simulink library "s2ss"  (R2015a)
settings: Solver=ode45  StartTime=0.0  StopTime=10.0  RelTol=1e-3
undefined symbols (not defined in the file or in its folder): AXI4, Lite
undefined symbols (not defined in the file): test
libraries: xbsIndex_r4 x92, s2ss x4
settings Model: Creator=ACS  LastModifiedBy=ACS

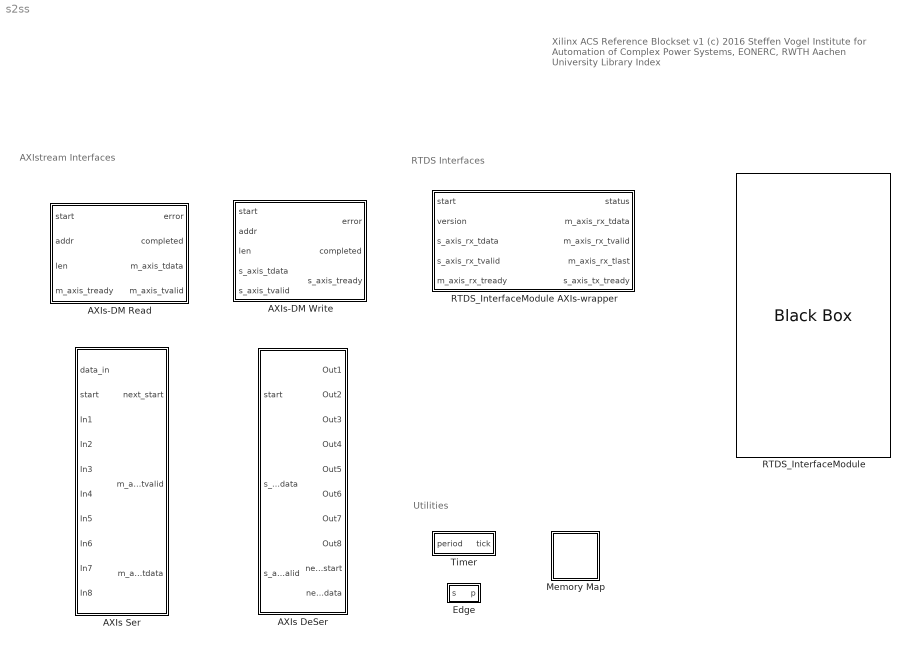
== system s2ss ==
  note: RTDS Interfaces
  note: AXIstream Interfaces
  note: Utilities
  note: Xilinx  ACS Reference Blockset v1
      | (c) 2016 Steffen Vogel
      | Institute for Automation of Complex Power Systems,
      | EONERC, RWTH Aachen University
      |
      | Library Index
  AXIs DeSer : Subsystem  mask(De-Serializing data to AXI-Steram){}
  AXIs Ser : Subsystem  mask(Serializing data to AXI-Steram){}
  AXIs-DM Read : Subsystem  mask(AXI DataMover: MM2S){}
  AXIs-DM Write : Subsystem  mask(AXI DataMover: S2MM){}
  Edge : Subsystem  mask(Rising edge detector){}
  Memory Map : Subsystem  InitFcn=|  mask(S2SS Memory Map){version=1.0, author=Steffen Vogel <stvogel@eonerc.rwth-aachen.de>, desc=System Generator Model, company_url=http://www.acs.eonerc.rwth-aachen.de, vendor=acs.eonerc.rwth-aachen.de, vendor_display_name=Institute for Automation of Complex Power Systems, EONERC, RWTH Aachen University, MaskMapDescription=test, map=[], created=[]}
      | map = xsg_memory_map();
      | %ts = floor(java.lang.System.currentTimeMillis / 1000);
      | 
      | set_param(gcb, 'map', mat2str(map));
      | %set_param(gcb, 'created', int2str(ts));
      mask prompts: desc "Description"; company_url "Company URL"; vendor_display_name "Vendor Display Name"
      mask help:
      | - This ROM contains a encoded memory map of all
      | Gateway In / Out blocks with an AXI4-Lite interface implementation.
      |
      | - The memory map is encoded in the function xsg_memory_map().
      |
      | - The CPU has to read the memory map word by word by using control
      |   registers 'map_addr' and 'map_data':
      |      1. Write address to 0x0 (map_addr)
      |      2. Read word from 0x4 (map_data)
      |      3. Increment address by 1 and start from 1
      |      4. Stop if word == 0xDEADBABE
      mask init:
      | set_param(gcb, 'MaskMapDescription', 'test');
      mask DialogControl DescTextMapVar Prompt: %<MaskMapDescription>
      mask Display:
      | color = [ hex2dec('FF') hex2dec('19') hex2dec('19') ] ./ 255;
      | 
      | patch([ 0 1 1 0 ], [ 0 0 0.2 0.2 ], color);
      | patch([ 0 1 1 0 ], [ 0.4 0.4 0.6 0.6 ], color);
      | patch([ 0 1 1 0 ], [ 0.8 0.8 1 1 ], color);
  RTDS_InterfaceModule : xbsIndex_r4/Black Box  init_code=RTDS_InterfaceModule_config  sim_method=ISE Simulator  verbose=off  block_type=blackbox2
  RTDS_InterfaceModule AXIs-wrapper : Subsystem  mask(AXI-Stream wrapper for RTDS_InterfaceModule blackbox){}
      mask Display: image(imread('logos/rtds.png'), [ 0.3 0.5 0.4 0.4 ])
  Timer : Subsystem  mask(Generate ticks every period cycles){}

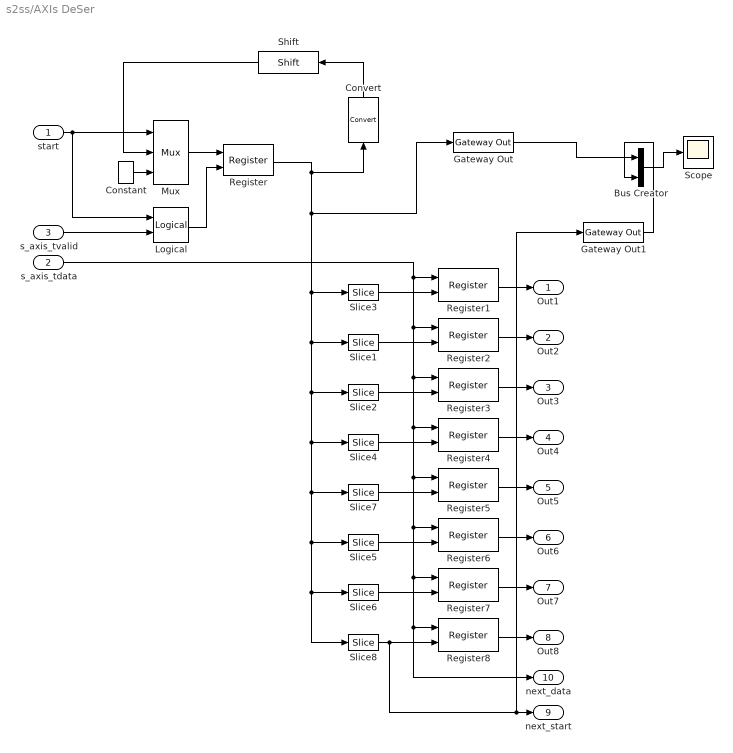
== system s2ss/AXIs DeSer ==
  start : Inport
  s_axis_tdata : Inport  Port=2
  s_axis_tvalid : Inport  Port=3
  Bus Creator : BusCreator  Inputs=2
  Constant : xbsIndex_r4/Constant  const=1  gui_display_data_type=Fixed-point  arith_type=Unsigned  n_bits=8  bin_pt=0  preci_type=Single  exp_width=8  frac_width=24  explicit_period=off  period=1  equ=P=C  opselect=C  inp2=PCIN>>17  opr=+  inp1=P  carry=CIN  dbl_ovrd=off  block_type=constant
  Convert : xbsIndex_r4/Convert  gui_display_data_type=Fixed-point  arith_type="Signed  (2's comp)"  n_bits=8  bin_pt=0  float_type=Single  exp_bits=8  fraction_bits=24  quantization=Truncate  overflow=Wrap  en=off  latency=0  pipeline=off  dbl_ovrd=off  block_type=convert
  Gateway Out : xbsIndex_r4/Gateway Out  inherit_from_input=off  hdl_port=on  rows=1  columns=1  UseAsDAC=off  DACChannel='1'  interface=None  automatic_assignment=on  address_offset=hex2dec('00')  intf_name=''  intf_description=''  timing_constraint=None  locs_specified=off  LOCs={}  io_standard={}  block_type=gatewayout
  Gateway Out1 : xbsIndex_r4/Gateway Out  inherit_from_input=off  hdl_port=on  rows=1  columns=1  UseAsDAC=off  DACChannel='1'  interface=None  automatic_assignment=on  address_offset=hex2dec('00')  intf_name=''  intf_description=''  timing_constraint=None  locs_specified=off  LOCs={}  io_standard={}  block_type=gatewayout
  Logical : xbsIndex_r4/Logical  logical_function=OR  inputs=2  en=off  latency=0  precision=Full  arith_type=Unsigned  n_bits=16  bin_pt=0  align_bp=on  dbl_ovrd=off  block_type=logical
  Mux : xbsIndex_r4/Mux  inputs=2  en=off  latency=0  precision=User Defined  arith_type=Unsigned  n_bits=8  bin_pt=0  quantization=Truncate  overflow=Wrap  dbl_ovrd=off  block_type=mux
  Register : xbsIndex_r4/Register  init=0  rst=off  en=on  dbl_ovrd=off  block_type=register
  Register{1..8} (8 alike) : xbsIndex_r4/Register  init=1  rst=off  en=on  dbl_ovrd=off  block_type=register
  Scope : Scope
  Shift : xbsIndex_r4/Shift  shift_dir=Left  shift_bits=1  en=off  latency=0  precision=Full  arith_type="Signed  (2's comp)"  n_bits=16  bin_pt=14  quantization=Truncate  overflow=Wrap  dbl_ovrd=off  block_type=shift
  Slice1 : xbsIndex_r4/Slice  nbits=1  boolean_output=on  mode=Lower Bit Location + Width  bit1=0  base1=MSB of Input  bit0=1  base0=LSB of Input  dbl_ovrd=off  block_type=slice
  Slice2 : xbsIndex_r4/Slice  nbits=1  boolean_output=on  mode=Lower Bit Location + Width  bit1=0  base1=MSB of Input  bit0=2  base0=LSB of Input  dbl_ovrd=off  block_type=slice
  Slice3 : xbsIndex_r4/Slice  nbits=1  boolean_output=on  mode=Lower Bit Location + Width  bit1=0  base1=MSB of Input  bit0=0  base0=LSB of Input  dbl_ovrd=off  block_type=slice
  Slice4 : xbsIndex_r4/Slice  nbits=1  boolean_output=on  mode=Lower Bit Location + Width  bit1=0  base1=MSB of Input  bit0=3  base0=LSB of Input  dbl_ovrd=off  block_type=slice
  Slice5 : xbsIndex_r4/Slice  nbits=1  boolean_output=on  mode=Lower Bit Location + Width  bit1=0  base1=MSB of Input  bit0=5  base0=LSB of Input  dbl_ovrd=off  block_type=slice
  Slice6 : xbsIndex_r4/Slice  nbits=1  boolean_output=on  mode=Lower Bit Location + Width  bit1=0  base1=MSB of Input  bit0=6  base0=LSB of Input  dbl_ovrd=off  block_type=slice
  Slice7 : xbsIndex_r4/Slice  nbits=1  boolean_output=on  mode=Lower Bit Location + Width  bit1=0  base1=MSB of Input  bit0=4  base0=LSB of Input  dbl_ovrd=off  block_type=slice
  Slice8 : xbsIndex_r4/Slice  nbits=1  boolean_output=on  mode=Lower Bit Location + Width  bit1=0  base1=MSB of Input  bit0=7  base0=LSB of Input  dbl_ovrd=off  block_type=slice
  Out1 : Outport
  Out2 : Outport  Port=2
  Out3 : Outport  Port=3
  Out4 : Outport  Port=4
  Out5 : Outport  Port=5
  Out6 : Outport  Port=6
  Out7 : Outport  Port=7
  Out8 : Outport  Port=8
  next_start : Outport  Port=9
  next_data : Outport  Port=10
  wires:
  Gateway Out1/1 -> Bus Creator/2
  Gateway Out/1 -> Bus Creator/1
  Bus Creator/1 -> Scope/1
  Shift/1 -> Mux/2
  Constant/1 -> Mux/3
  Logical/1 -> Register/2
  s_axis_tvalid/1 -> Logical/2
  Mux/1 -> Register/1
  start/1 -> Mux/1, Logical/1
  Convert/1 -> Shift/1
  Register8/1 -> Out8/1
  Slice8/1 -> next_start/1, Gateway Out1/1, Register8/2
  Register7/1 -> Out7/1
  Slice6/1 -> Register7/2
  Register6/1 -> Out6/1
  Slice5/1 -> Register6/2
  Register5/1 -> Out5/1
  Slice7/1 -> Register5/2
  Register4/1 -> Out4/1
  Slice4/1 -> Register4/2
  Register3/1 -> Out3/1
  Slice2/1 -> Register3/2
  Register2/1 -> Out2/1
  Slice1/1 -> Register2/2
  Register1/1 -> Out1/1
  s_axis_tdata/1 -> Register1/1, Register8/1, next_data/1, Register7/1, Register6/1, Register5/1, Register4/1, Register3/1, Register2/1
  Register/1 -> Convert/1, Slice3/1, Slice1/1, Slice2/1, Slice4/1, Slice7/1, Slice5/1, Slice6/1, Slice8/1, Gateway Out/1
  Slice3/1 -> Register1/2

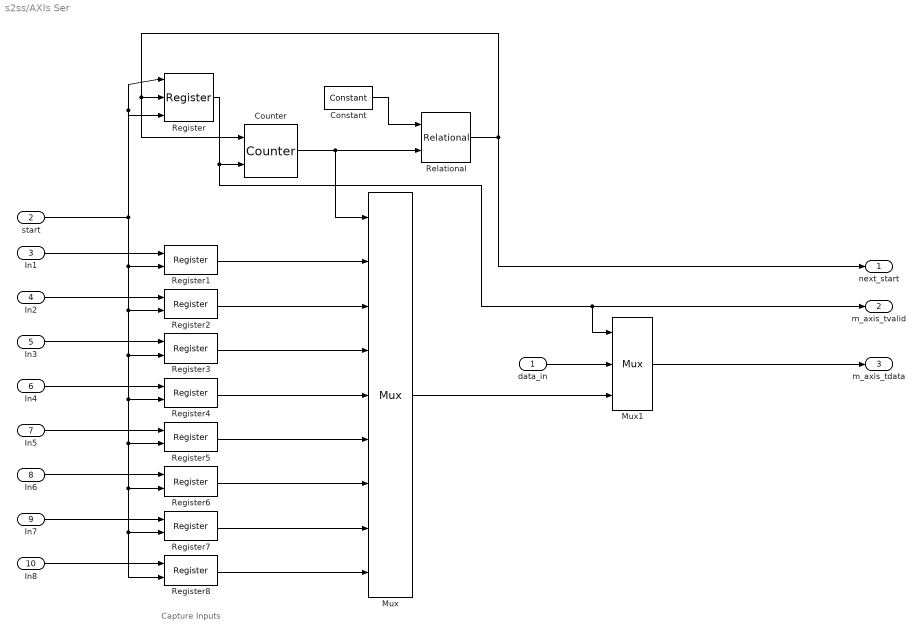
== system s2ss/AXIs Ser ==
  note: Capture Inputs
  data_in : Inport
  start : Inport  Port=2
  In1 : Inport  Port=3
  In2 : Inport  Port=4
  In3 : Inport  Port=5
  In4 : Inport  Port=6
  In5 : Inport  Port=7
  In6 : Inport  Port=8
  In7 : Inport  Port=9
  In8 : Inport  Port=10
  Constant : xbsIndex_r4/Constant  const=7  gui_display_data_type=Fixed-point  arith_type=Unsigned  n_bits=3  bin_pt=0  preci_type=Single  exp_width=8  frac_width=24  explicit_period=off  period=1  equ=P=C  opselect=C  inp2=PCIN>>17  opr=+  inp1=P  carry=CIN  dbl_ovrd=off  block_type=constant
  Counter : xbsIndex_r4/Counter  cnt_type=Free Running  cnt_to=Inf  operation=Up  start_count=0  cnt_by_val=1  arith_type=Unsigned  n_bits=3  bin_pt=0  load_pin=off  rst=on  en=on  explicit_period=on  period=1  use_behavioral_HDL=off  implementation=Fabric  dbl_ovrd=off  block_type=counter
  Mux : xbsIndex_r4/Mux  inputs=8  en=off  latency=0  precision=Full  arith_type=Unsigned  n_bits=16  bin_pt=14  quantization=Truncate  overflow=Wrap  dbl_ovrd=off  block_type=mux
  Mux1 : xbsIndex_r4/Mux  inputs=2  en=off  latency=1  precision=Full  arith_type=Unsigned  n_bits=16  bin_pt=14  quantization=Truncate  overflow=Wrap  dbl_ovrd=off  block_type=mux
  Register : xbsIndex_r4/Register  init=0  rst=on  en=on  dbl_ovrd=off  block_type=register
  Register{1..8} (8 alike) : xbsIndex_r4/Register  init=1  rst=off  en=on  dbl_ovrd=off  block_type=register
  Relational : xbsIndex_r4/Relational  mode=a=b  op_type=Bool  en=off  latency=0  dbl_ovrd=off  block_type=relational
  next_start : Outport
  "m_axis_tvalid " : Outport  Port=2
  m_axis_tdata : Outport  Port=3
  wires:
  data_in/1 -> Mux1/2
  Mux1/1 -> m_axis_tdata/1
  Register/1 -> "m_axis_tvalid "/1, Mux1/1, Counter/2
  Relational/1 -> next_start/1, Register/2, Counter/1
  Constant/1 -> Relational/1
  Register8/1 -> Mux/9
  Register7/1 -> Mux/8
  Register6/1 -> Mux/7
  Register5/1 -> Mux/6
  Register4/1 -> Mux/5
  Register3/1 -> Mux/4
  Register2/1 -> Mux/3
  Register1/1 -> Mux/2
  Counter/1 -> Relational/2, Mux/1
  Mux/1 -> Mux1/3
  In8/1 -> Register8/1
  In7/1 -> Register7/1
  In6/1 -> Register6/1
  In5/1 -> Register5/1
  In4/1 -> Register4/1
  In1/1 -> Register1/1
  In2/1 -> Register2/1
  In3/1 -> Register3/1
  start/1 -> Register1/2, Register2/2, Register3/2, Register4/2, Register5/2, Register6/2, Register7/2, Register8/2, Register/1, Register/3

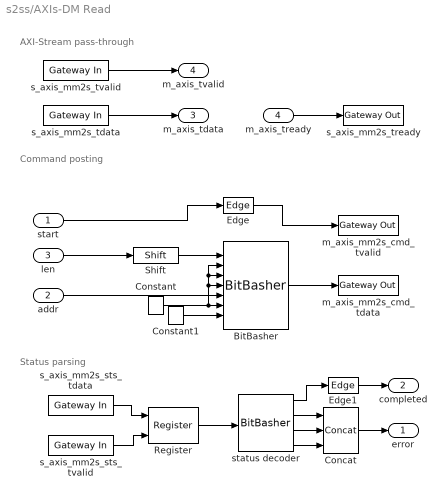
== system s2ss/AXIs-DM Read ==
  note: AXI-Stream pass-through
  note: Command posting
  note: Status parsing
  start : Inport
  addr : Inport  Port=2
  len : Inport  Port=3
  m_axis_tready : Inport  Port=4
  "BitBasher " : xbsIndex_r4/BitBasher  bitexpr=cmd={4'h0,tag[3:0],saddr[31:0],drr[0],eof[0],dsa[5:0],type[0],btt[22:0]}  display_expr=off  sr_1=cmd  arith_type1=Unsigned  bin_pt1=0  sr_2=2  arith_type2=Unsigned  bin_pt2=0  sr_3=3  arith_type3=Unsigned  bin_pt3=0  sr_4=4  arith_type4=Unsigned  bin_pt4=0  dbl_ovrd=off  block_type=bitbasher
  Concat : xbsIndex_r4/Concat  num_inputs=3  dbl_ovrd=off  block_type=concat
  Constant : xbsIndex_r4/Constant  const=0  gui_display_data_type=Fixed-point  arith_type=Unsigned  n_bits=16  bin_pt=0  preci_type=Single  exp_width=8  frac_width=24  explicit_period=off  period=1  equ=P=C  opselect=C  inp2=PCIN>>17  opr=+  inp1=P  carry=CIN  dbl_ovrd=off  block_type=constant
  Constant1 : xbsIndex_r4/Constant  const=1  gui_display_data_type=Fixed-point  arith_type=Unsigned  n_bits=16  bin_pt=0  preci_type=Single  exp_width=8  frac_width=24  explicit_period=off  period=1  equ=P=C  opselect=C  inp2=PCIN>>17  opr=+  inp1=P  carry=CIN  dbl_ovrd=off  block_type=constant
  Edge : s2ss/Edge  SystemSampleTime=-1
  Edge1 : s2ss/Edge  SystemSampleTime=-1
  Register : xbsIndex_r4/Register  init=0  rst=off  en=on  dbl_ovrd=off  block_type=register
  Shift : xbsIndex_r4/Shift  shift_dir=Left  shift_bits=2  en=off  latency=0  precision=User Defined  arith_type=Unsigned  n_bits=23  bin_pt=0  quantization=Truncate  overflow=Wrap  dbl_ovrd=off  block_type=shift
  m_axis_mm2s_cmd_tdata : xbsIndex_r4/Gateway Out  inherit_from_input=off  hdl_port=on  rows=1  columns=1  UseAsDAC=off  DACChannel='1'  interface=None  automatic_assignment=on  address_offset=hex2dec('00')  intf_name=''  intf_description=''  timing_constraint=None  locs_specified=off  LOCs={}  io_standard={}  block_type=gatewayout
  m_axis_mm2s_cmd_tvalid : xbsIndex_r4/Gateway Out  inherit_from_input=off  hdl_port=on  rows=1  columns=1  UseAsDAC=off  DACChannel='1'  interface=None  automatic_assignment=on  address_offset=hex2dec('00')  intf_name=''  intf_description=''  timing_constraint=None  locs_specified=off  LOCs={}  io_standard={}  block_type=gatewayout
  s_axis_mm2s_sts_tdata : xbsIndex_r4/Gateway In  gui_display_data_type=Fixed-point  arith_type=Unsigned  n_bits=8  bin_pt=0  preci_type=Single  exp_width=8  frac_width=24  rows=1  columns=1  quantization=Truncate  overflow=Wrap  period=1  UseAsADC=off  ADCChannel='1'  interface=None  automatic_assignment=on  address_offset=hex2dec('00')  intf_name=''  intf_description=''  timing_constraint=None  locs_specified=off  LOCs={}  io_standard={}  inherit_from_input=off  hdl_port=on  dbl_ovrd=off  block_type=gatewayin
  s_axis_mm2s_sts_tvalid : xbsIndex_r4/Gateway In  gui_display_data_type=Boolean  arith_type=Boolean  n_bits=1  bin_pt=0  preci_type=Single  exp_width=8  frac_width=24  rows=1  columns=1  quantization="Round  (unbiased: +/- Inf)"  overflow=Saturate  period=1  UseAsADC=off  ADCChannel='1'  interface=None  automatic_assignment=on  address_offset=hex2dec('00')  intf_name=''  intf_description=''  timing_constraint=None  locs_specified=off  LOCs={}  io_standard={}  inherit_from_input=off  hdl_port=on  dbl_ovrd=off  block_type=gatewayin
  s_axis_mm2s_tdata : xbsIndex_r4/Gateway In  gui_display_data_type=Fixed-point  arith_type=Unsigned  n_bits=32  bin_pt=0  preci_type=Single  exp_width=8  frac_width=24  rows=1  columns=1  quantization=Truncate  overflow=Wrap  period=1  UseAsADC=off  ADCChannel='1'  interface=None  automatic_assignment=on  address_offset=hex2dec('00')  intf_name=''  intf_description=''  timing_constraint=None  locs_specified=off  LOCs={}  io_standard={}  inherit_from_input=off  hdl_port=on  dbl_ovrd=off  block_type=gatewayin
  s_axis_mm2s_tready : xbsIndex_r4/Gateway Out  inherit_from_input=off  hdl_port=on  rows=1  columns=1  UseAsDAC=off  DACChannel='1'  interface=None  automatic_assignment=on  address_offset=hex2dec('00')  intf_name=''  intf_description=''  timing_constraint=None  locs_specified=off  LOCs={}  io_standard={}  block_type=gatewayout
  s_axis_mm2s_tvalid : xbsIndex_r4/Gateway In  gui_display_data_type=Boolean  arith_type=Boolean  n_bits=16  bin_pt=14  preci_type=Single  exp_width=8  frac_width=24  rows=1  columns=1  quantization="Round  (unbiased: +/- Inf)"  overflow=Saturate  period=1  UseAsADC=off  ADCChannel='1'  interface=None  automatic_assignment=on  address_offset=hex2dec('00')  intf_name=''  intf_description=''  timing_constraint=None  locs_specified=off  LOCs={}  io_standard={}  inherit_from_input=off  hdl_port=on  dbl_ovrd=off  block_type=gatewayin
  status decoder : xbsIndex_r4/BitBasher  bitexpr=|  display_expr=off  sr_1=okay  arith_type1=Unsigned  bin_pt1=0  sr_2=slverr  arith_type2=Unsigned  bin_pt2=0  sr_3=decerr  arith_type3=Unsigned  bin_pt3=0  sr_4=interr  arith_type4=Unsigned  bin_pt4=0  dbl_ovrd=off  block_type=bitbasher
      | okay={sts[7]}
      | slverr={sts[6]}
      | decerr={sts[5]}
      | interr={sts[4]}
  error : Outport
  completed : Outport  Port=2
  m_axis_tdata : Outport  Port=3
  m_axis_tvalid : Outport  Port=4
  wires:
  Shift/1 -> "BitBasher "/1
  "BitBasher "/1 -> m_axis_mm2s_cmd_tdata/1
  s_axis_mm2s_sts_tdata/1 -> Register/1
  s_axis_mm2s_sts_tvalid/1 -> Register/2
  Register/1 -> status decoder/1
  status decoder/4 -> Concat/3
  Concat/1 -> error/1
  Edge/1 -> m_axis_mm2s_cmd_tvalid/1
  len/1 -> Shift/1
  start/1 -> Edge/1
  status decoder/3 -> Concat/2
  status decoder/2 -> Concat/1
  s_axis_mm2s_tvalid/1 -> m_axis_tvalid/1
  s_axis_mm2s_tdata/1 -> m_axis_tdata/1
  m_axis_tready/1 -> s_axis_mm2s_tready/1
  addr/1 -> "BitBasher "/5
  Constant/1 -> "BitBasher "/2, "BitBasher "/3, "BitBasher "/4, "BitBasher "/6
  status decoder/1 -> Edge1/1
  Edge1/1 -> completed/1
  Constant1/1 -> "BitBasher "/7

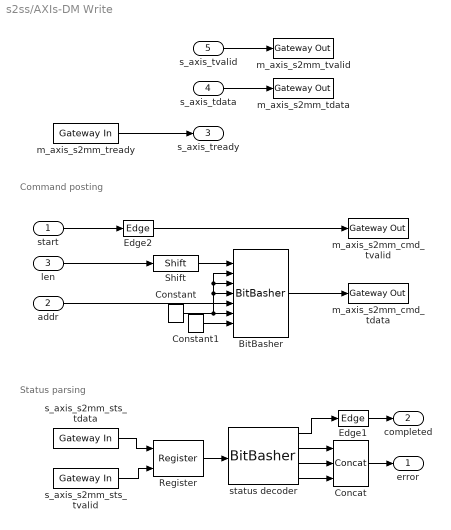
== system s2ss/AXIs-DM Write ==
  note: Command posting
  note: Status parsing
  start : Inport
  addr : Inport  Port=2
  len : Inport  Port=3
  s_axis_tdata : Inport  Port=4
  s_axis_tvalid : Inport  Port=5
  "BitBasher " : xbsIndex_r4/BitBasher  bitexpr=cmd={4'h0,tag[3:0],saddr[31:0],drr[0],eof[0],dsa[5:0],type[0],btt[22:0]}  display_expr=off  sr_1=cmd  arith_type1=Unsigned  bin_pt1=0  sr_2=2  arith_type2=Unsigned  bin_pt2=0  sr_3=3  arith_type3=Unsigned  bin_pt3=0  sr_4=4  arith_type4=Unsigned  bin_pt4=0  dbl_ovrd=off  block_type=bitbasher
  Concat : xbsIndex_r4/Concat  num_inputs=3  dbl_ovrd=off  block_type=concat
  Constant : xbsIndex_r4/Constant  const=0  gui_display_data_type=Fixed-point  arith_type=Unsigned  n_bits=16  bin_pt=0  preci_type=Single  exp_width=8  frac_width=24  explicit_period=off  period=1  equ=P=C  opselect=C  inp2=PCIN>>17  opr=+  inp1=P  carry=CIN  dbl_ovrd=off  block_type=constant
  Constant1 : xbsIndex_r4/Constant  const=1  gui_display_data_type=Fixed-point  arith_type=Unsigned  n_bits=16  bin_pt=0  preci_type=Single  exp_width=8  frac_width=24  explicit_period=off  period=1  equ=P=C  opselect=C  inp2=PCIN>>17  opr=+  inp1=P  carry=CIN  dbl_ovrd=off  block_type=constant
  Edge1 : s2ss/Edge  SystemSampleTime=-1
  Edge2 : s2ss/Edge  SystemSampleTime=-1
  Register : xbsIndex_r4/Register  init=0  rst=off  en=on  dbl_ovrd=off  block_type=register
  Shift : xbsIndex_r4/Shift  shift_dir=Left  shift_bits=2  en=off  latency=0  precision=User Defined  arith_type=Unsigned  n_bits=23  bin_pt=0  quantization=Truncate  overflow=Wrap  dbl_ovrd=off  block_type=shift
  m_axis_s2mm_cmd_tdata : xbsIndex_r4/Gateway Out  inherit_from_input=off  hdl_port=on  rows=1  columns=1  UseAsDAC=off  DACChannel='1'  interface=None  automatic_assignment=on  address_offset=hex2dec('00')  intf_name=''  intf_description=''  timing_constraint=None  locs_specified=off  LOCs={}  io_standard={}  block_type=gatewayout
  m_axis_s2mm_cmd_tvalid : xbsIndex_r4/Gateway Out  inherit_from_input=off  hdl_port=on  rows=1  columns=1  UseAsDAC=off  DACChannel='1'  interface=None  automatic_assignment=on  address_offset=hex2dec('00')  intf_name=''  intf_description=''  timing_constraint=None  locs_specified=off  LOCs={}  io_standard={}  block_type=gatewayout
  m_axis_s2mm_tdata : xbsIndex_r4/Gateway Out  inherit_from_input=off  hdl_port=on  rows=1  columns=1  UseAsDAC=off  DACChannel='1'  interface=None  automatic_assignment=on  address_offset=hex2dec('00')  intf_name=''  intf_description=''  timing_constraint=None  locs_specified=off  LOCs={}  io_standard={}  block_type=gatewayout
  m_axis_s2mm_tready : xbsIndex_r4/Gateway In  gui_display_data_type=Boolean  arith_type=Boolean  n_bits=8  bin_pt=0  preci_type=Single  exp_width=8  frac_width=24  rows=1  columns=1  quantization=Truncate  overflow=Wrap  period=1  UseAsADC=off  ADCChannel='1'  interface=None  automatic_assignment=on  address_offset=hex2dec('00')  intf_name=''  intf_description=''  timing_constraint=None  locs_specified=off  LOCs={}  io_standard={}  inherit_from_input=off  hdl_port=on  dbl_ovrd=off  block_type=gatewayin
  m_axis_s2mm_tvalid : xbsIndex_r4/Gateway Out  inherit_from_input=off  hdl_port=on  rows=1  columns=1  UseAsDAC=off  DACChannel='1'  interface=None  automatic_assignment=on  address_offset=hex2dec('00')  intf_name=''  intf_description=''  timing_constraint=None  locs_specified=off  LOCs={}  io_standard={}  block_type=gatewayout
  s_axis_s2mm_sts_tdata : xbsIndex_r4/Gateway In  gui_display_data_type=Fixed-point  arith_type=Unsigned  n_bits=8  bin_pt=0  preci_type=Single  exp_width=8  frac_width=24  rows=1  columns=1  quantization=Truncate  overflow=Wrap  period=1  UseAsADC=off  ADCChannel='1'  interface=None  automatic_assignment=on  address_offset=hex2dec('00')  intf_name=''  intf_description=''  timing_constraint=None  locs_specified=off  LOCs={}  io_standard={}  inherit_from_input=off  hdl_port=on  dbl_ovrd=off  block_type=gatewayin
  s_axis_s2mm_sts_tvalid : xbsIndex_r4/Gateway In  gui_display_data_type=Boolean  arith_type=Boolean  n_bits=16  bin_pt=14  preci_type=Single  exp_width=8  frac_width=24  rows=1  columns=1  quantization="Round  (unbiased: +/- Inf)"  overflow=Saturate  period=1  UseAsADC=off  ADCChannel='1'  interface=None  automatic_assignment=on  address_offset=hex2dec('00')  intf_name=''  intf_description=''  timing_constraint=None  locs_specified=off  LOCs={}  io_standard={}  inherit_from_input=off  hdl_port=on  dbl_ovrd=off  block_type=gatewayin
  status decoder : xbsIndex_r4/BitBasher  bitexpr=|  display_expr=off  sr_1=okay  arith_type1=Unsigned  bin_pt1=0  sr_2=slverr  arith_type2=Unsigned  bin_pt2=0  sr_3=decerr  arith_type3=Unsigned  bin_pt3=0  sr_4=interr  arith_type4=Unsigned  bin_pt4=0  dbl_ovrd=off  block_type=bitbasher
      | okay={sts[7]}
      | slverr={sts[6]}
      | decerr={sts[5]}
      | interr={sts[4]}
  error : Outport
  completed : Outport  Port=2
  s_axis_tready : Outport  Port=3
  wires:
  addr/1 -> "BitBasher "/5
  Shift/1 -> "BitBasher "/1
  "BitBasher "/1 -> m_axis_s2mm_cmd_tdata/1
  s_axis_s2mm_sts_tdata/1 -> Register/1
  s_axis_s2mm_sts_tvalid/1 -> Register/2
  Register/1 -> status decoder/1
  status decoder/4 -> Concat/3
  Concat/1 -> error/1
  start/1 -> Edge2/1
  s_axis_tvalid/1 -> m_axis_s2mm_tvalid/1
  s_axis_tdata/1 -> m_axis_s2mm_tdata/1
  len/1 -> Shift/1
  Edge2/1 -> m_axis_s2mm_cmd_tvalid/1
  m_axis_s2mm_tready/1 -> s_axis_tready/1
  status decoder/3 -> Concat/2
  status decoder/2 -> Concat/1
  status decoder/1 -> Edge1/1
  Constant/1 -> "BitBasher "/6, "BitBasher "/4, "BitBasher "/3, "BitBasher "/2
  Edge1/1 -> completed/1
  Constant1/1 -> "BitBasher "/7

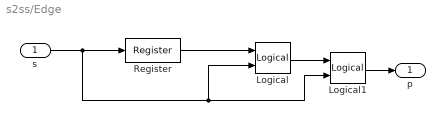
== system s2ss/Edge ==
  s : Inport
  Logical : xbsIndex_r4/Logical  logical_function=XOR  inputs=2  en=off  latency=0  precision=Full  arith_type=Unsigned  n_bits=16  bin_pt=0  align_bp=on  dbl_ovrd=off  block_type=logical
  Logical1 : xbsIndex_r4/Logical  logical_function=AND  inputs=2  en=off  latency=0  precision=Full  arith_type=Unsigned  n_bits=16  bin_pt=0  align_bp=on  dbl_ovrd=off  block_type=logical
  Register : xbsIndex_r4/Register  init=0  rst=off  en=off  dbl_ovrd=off  block_type=register
  p : Outport
  wires:
  s/1 -> Logical/2, Logical1/2, Register/1
  Register/1 -> Logical/1
  Logical1/1 -> p/1
  Logical/1 -> Logical1/1

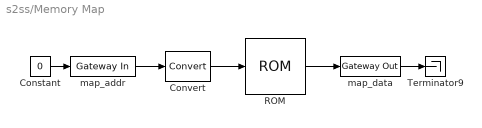
== system s2ss/Memory Map ==
  Constant : Constant  Value=0
  Convert : xbsIndex_r4/Convert  gui_display_data_type=Fixed-point  arith_type=Unsigned  n_bits=ceil(log2(length(map)))  bin_pt=0  float_type=Single  exp_bits=8  fraction_bits=24  quantization=Truncate  overflow=Wrap  en=off  latency=1  pipeline=off  dbl_ovrd=off  block_type=convert
  ROM : xbsIndex_r4/ROM  depth=length(map)  initVector=map  distributed_mem=Block RAM  rst=off  init_reg=0  en=off  latency=1  gui_display_data_type=Fixed-point  arith_type=Unsigned  n_bits=32  bin_pt=0  preci_type=Single  exp_width=8  frac_width=24  optimize=Area  use_rpm=on  dbl_ovrd=off  block_type=sprom
  Terminator9 : Terminator
  map_addr : xbsIndex_r4/Gateway In  gui_display_data_type=Fixed-point  arith_type=Unsigned  n_bits=32  bin_pt=0  preci_type=Single  exp_width=8  frac_width=24  rows=1  columns=1  quantization=Truncate  overflow=Wrap  period=1  UseAsADC=off  ADCChannel='1'  interface=AXI4-Lite  automatic_assignment=off  address_offset=hex2dec('00')  intf_name=''  intf_description=''  timing_constraint=None  locs_specified=off  LOCs={}  io_standard={}  inherit_from_input=off  hdl_port=on  dbl_ovrd=off  block_type=gatewayin
  map_data : xbsIndex_r4/Gateway Out  inherit_from_input=off  hdl_port=on  rows=1  columns=1  UseAsDAC=off  DACChannel='1'  interface=AXI4-Lite  automatic_assignment=off  address_offset=hex2dec('04')  intf_name=''  intf_description=''  timing_constraint=None  locs_specified=off  LOCs={}  io_standard={}  block_type=gatewayout
  wires:
  ROM/1 -> map_data/1
  map_addr/1 -> Convert/1
  Convert/1 -> ROM/1
  map_data/1 -> Terminator9/1
  Constant/1 -> map_addr/1

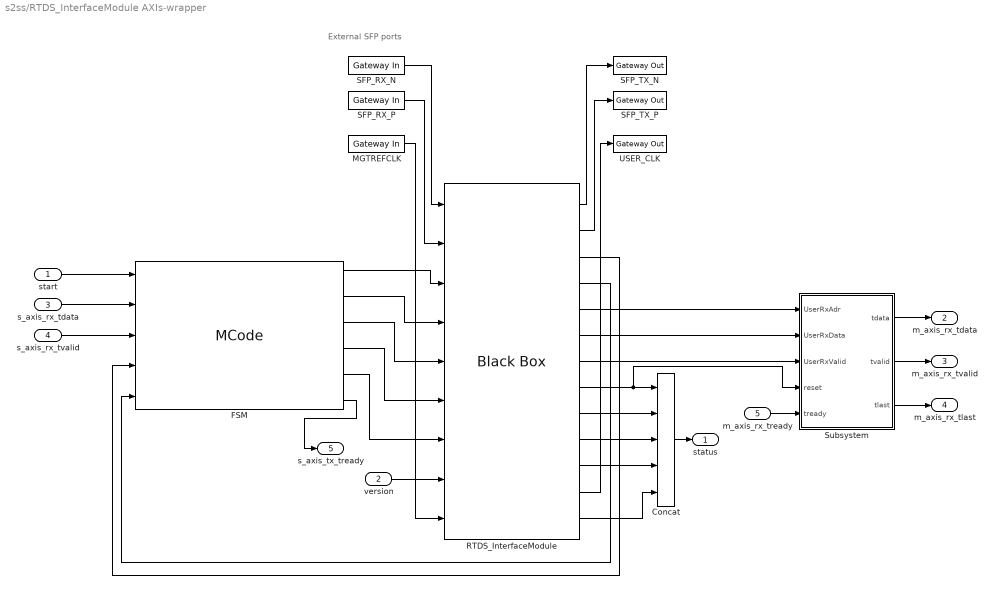
== system s2ss/RTDS_InterfaceModule AXIs-wrapper ==
  note: External SFP ports
  start : Inport
  version : Inport  Port=2
  s_axis_rx_tdata : Inport  Port=3
  s_axis_rx_tvalid : Inport  Port=4
  m_axis_rx_tready : Inport  Port=5
  Concat : xbsIndex_r4/Concat  num_inputs=5  dbl_ovrd=off  block_type=concat
  FSM : xbsIndex_r4/MCode  mfname=RTDS_InferfaceModule_fsm  explicit_period=off  period=1  inputsTable={'boundInpExpr'=>['','','',''],'inputs'=>['start','NbValues','UserTxFull','UserTxInProgress']}  outputsTable={'outputs'=>['UserTxAdr','UserTxData','UserTxWr','UserLockBank','UserFreeBank'],'suppressOut'=>['off','off','off','off','off']}  enable_stdout=off  enable_debug=off  suppress_output=on  defparams={}  hide_port_list={}  dbl_ovrd=off  block_type=mcode
  MGTREFCLK : xbsIndex_r4/Gateway In  gui_display_data_type=Boolean  arith_type=Boolean  n_bits=16  bin_pt=14  preci_type=Single  exp_width=8  frac_width=24  rows=1  columns=1  quantization="Round  (unbiased: +/- Inf)"  overflow=Saturate  period=1  UseAsADC=off  ADCChannel='1'  interface=None  automatic_assignment=on  address_offset=hex2dec('00')  intf_name=''  intf_description=''  timing_constraint=None  locs_specified=off  LOCs={}  io_standard={}  inherit_from_input=off  hdl_port=on  dbl_ovrd=off  block_type=gatewayin
  RTDS_InterfaceModule : xbsIndex_r4/Black Box  init_code=RTDS_InterfaceModule_config  sim_method=ISE Simulator  verbose=off  block_type=blackbox2
  SFP_RX_N : xbsIndex_r4/Gateway In  gui_display_data_type=Boolean  arith_type=Boolean  n_bits=1  bin_pt=0  preci_type=Single  exp_width=8  frac_width=24  rows=1  columns=1  quantization="Round  (unbiased: +/- Inf)"  overflow=Saturate  period=1  UseAsADC=off  ADCChannel='1'  interface=None  automatic_assignment=on  address_offset=hex2dec('00')  intf_name=''  intf_description=''  timing_constraint=None  locs_specified=off  LOCs={}  io_standard={}  inherit_from_input=off  hdl_port=on  dbl_ovrd=off  block_type=gatewayin
  SFP_RX_P : xbsIndex_r4/Gateway In  gui_display_data_type=Boolean  arith_type=Boolean  n_bits=16  bin_pt=14  preci_type=Single  exp_width=8  frac_width=24  rows=1  columns=1  quantization="Round  (unbiased: +/- Inf)"  overflow=Saturate  period=1  UseAsADC=off  ADCChannel='1'  interface=None  automatic_assignment=on  address_offset=hex2dec('00')  intf_name=''  intf_description=''  timing_constraint=None  locs_specified=off  LOCs={}  io_standard={}  inherit_from_input=off  hdl_port=on  dbl_ovrd=off  block_type=gatewayin
  SFP_TX_N : xbsIndex_r4/Gateway Out  inherit_from_input=off  hdl_port=on  rows=1  columns=1  UseAsDAC=off  DACChannel='1'  interface=None  automatic_assignment=on  address_offset=hex2dec('00')  intf_name=''  intf_description=''  timing_constraint=None  locs_specified=off  LOCs={}  io_standard={}  block_type=gatewayout
  "SFP_TX_P " : xbsIndex_r4/Gateway Out  inherit_from_input=off  hdl_port=on  rows=1  columns=1  UseAsDAC=off  DACChannel='1'  interface=None  automatic_assignment=on  address_offset=hex2dec('00')  intf_name=''  intf_description=''  timing_constraint=None  locs_specified=off  LOCs={}  io_standard={}  block_type=gatewayout
  Subsystem : Subsystem
  USER_CLK : xbsIndex_r4/Gateway Out  inherit_from_input=off  hdl_port=on  rows=1  columns=1  UseAsDAC=off  DACChannel='1'  interface=None  automatic_assignment=on  address_offset=hex2dec('00')  intf_name=''  intf_description=''  timing_constraint=None  locs_specified=off  LOCs={}  io_standard={}  block_type=gatewayout
  status : Outport
  m_axis_rx_tdata : Outport  Port=2
  m_axis_rx_tvalid : Outport  Port=3
  m_axis_rx_tlast : Outport  Port=4
  s_axis_tx_tready : Outport  Port=5
  wires:
  version/1 -> RTDS_InterfaceModule/8
  RTDS_InterfaceModule/4 -> FSM/5
  RTDS_InterfaceModule/13 -> Concat/5
  RTDS_InterfaceModule/10 -> Concat/3
  RTDS_InterfaceModule/11 -> Concat/4
  RTDS_InterfaceModule/9 -> Concat/2
  RTDS_InterfaceModule/8 -> Subsystem/4(reset), Concat/1
  RTDS_InterfaceModule/12 -> USER_CLK/1
  SFP_RX_N/1 -> RTDS_InterfaceModule/1
  SFP_RX_P/1 -> RTDS_InterfaceModule/2
  MGTREFCLK/1 -> RTDS_InterfaceModule/9
  RTDS_InterfaceModule/1 -> SFP_TX_N/1
  RTDS_InterfaceModule/2 -> "SFP_TX_P "/1
  FSM/3 -> RTDS_InterfaceModule/5
  FSM/1 -> RTDS_InterfaceModule/3
  FSM/4 -> RTDS_InterfaceModule/6
  start/1 -> FSM/1
  FSM/2 -> RTDS_InterfaceModule/4
  FSM/5 -> RTDS_InterfaceModule/7
  RTDS_InterfaceModule/3 -> FSM/4
  Concat/1 -> status/1
  FSM/6 -> s_axis_tx_tready/1
  RTDS_InterfaceModule/5 -> Subsystem/1(UserRxAdr)
  RTDS_InterfaceModule/6 -> Subsystem/2(UserRxData)
  RTDS_InterfaceModule/7 -> Subsystem/3(UserRxValid)
  Subsystem/1(tdata) -> m_axis_rx_tdata/1
  Subsystem/2(tvalid) -> m_axis_rx_tvalid/1
  m_axis_rx_tready/1 -> Subsystem/5(tready)
  Subsystem/3(tlast) -> m_axis_rx_tlast/1
  s_axis_rx_tdata/1 -> FSM/2
  s_axis_rx_tvalid/1 -> FSM/3

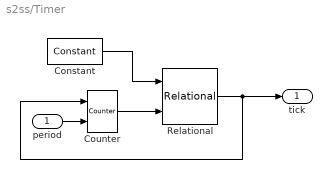
== system s2ss/Timer ==
  period : Inport
  Constant : xbsIndex_r4/Constant  const=1  gui_display_data_type=Fixed-point  arith_type=Signed (2's comp)  n_bits=32  bin_pt=0  preci_type=Single  exp_width=8  frac_width=24  explicit_period=off  period=1  equ=P=C  opselect=C  inp2=PCIN>>17  opr=+  inp1=P  carry=CIN  dbl_ovrd=off  block_type=constant
  Counter : xbsIndex_r4/Counter  cnt_type=Free Running  cnt_to=Inf  operation=Down  start_count=1  cnt_by_val=1  arith_type=Unsigned  n_bits=32  bin_pt=0  load_pin=on  rst=off  en=off  explicit_period=on  period=1  use_behavioral_HDL=off  implementation=Fabric  dbl_ovrd=off  block_type=counter
  Relational : xbsIndex_r4/Relational  mode=a=b  op_type=Bool  en=off  latency=0  dbl_ovrd=off  block_type=relational
  tick : Outport
  wires:
  Counter/1 -> Relational/2
  Relational/1 -> Counter/1, tick/1
  period/1 -> Counter/2
  Constant/1 -> Relational/1

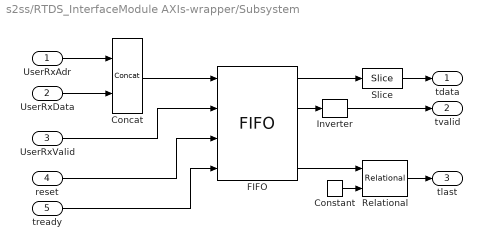
== system s2ss/RTDS_InterfaceModule AXIs-wrapper/Subsystem ==
  UserRxAdr : Inport
  UserRxData : Inport  Port=2
  UserRxValid : Inport  Port=3
  reset : Inport  Port=4
  tready : Inport  Port=5
  Concat : xbsIndex_r4/Concat  num_inputs=2  dbl_ovrd=off  block_type=concat
  Constant : xbsIndex_r4/Constant  const=1.0  gui_display_data_type=Fixed-point  arith_type=Signed (2's comp)  n_bits=16  bin_pt=14  preci_type=Single  exp_width=8  frac_width=24  explicit_period=off  period=1  equ=P=C  opselect=C  inp2=PCIN>>17  opr=+  inp1=P  carry=CIN  dbl_ovrd=off  block_type=constant
  FIFO : xbsIndex_r4/FIFO  mem_type=Block RAM  performance_options=Standard_FIFO  embedded_registers=off  depth=64  percent_nbits=1  rst=off  rst_latency=1  en=on  use_dcount=on  use_percent_full_port=off  use_almost_empty=off  almost_empty_thresh=2  use_almost_full=off  almost_full_thresh=14  explicit_period=off  dbl_ovrd=off  block_type=fifo
  Inverter : xbsIndex_r4/Inverter  en=off  latency=0  dbl_ovrd=off  block_type=inv
  Relational : xbsIndex_r4/Relational  mode=a=b  op_type=Bool  en=off  latency=0  dbl_ovrd=off  block_type=relational
  Slice : xbsIndex_r4/Slice  nbits=32  boolean_output=off  mode=Lower Bit Location + Width  bit1=0  base1=MSB of Input  bit0=0  base0=LSB of Input  dbl_ovrd=off  block_type=slice
  tdata : Outport
  tvalid : Outport  Port=2
  tlast : Outport  Port=3
  wires:
  UserRxAdr/1 -> Concat/1
  UserRxData/1 -> Concat/2
  Concat/1 -> FIFO/1
  UserRxValid/1 -> FIFO/2
  FIFO/1 -> Slice/1
  FIFO/2 -> Inverter/1
  Inverter/1 -> tvalid/1
  reset/1 -> FIFO/3
  tready/1 -> FIFO/4
  Slice/1 -> tdata/1
  FIFO/4 -> Relational/1
  Constant/1 -> Relational/2
  Relational/1 -> tlast/1
